simulink model "solics_inverter_model_updated"  (R2024a)
settings: Solver=VariableStepAuto  StartTime=0.0  StopTime=1  RelTol=1e-3
libraries: spsSeriesRLCBranchLib x7, spsIGBTLib x5, spsVoltageMeasurementLib x4, spsCurrentMeasurementLib x3, spsGroundLib x2, spsDiodeLib x1, spsPVArrayLib x1, spsPWMGeneratorDCDCLib x1, spsTriangleGeneratorLib x1, spspowerguiLib x1
settings Model: Creator=dogba  LastModifiedBy=dogba

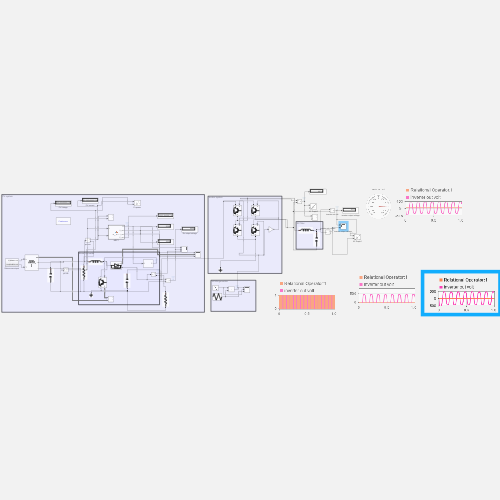
[thumbnail: Simulink's stored preview of the top-level diagram]
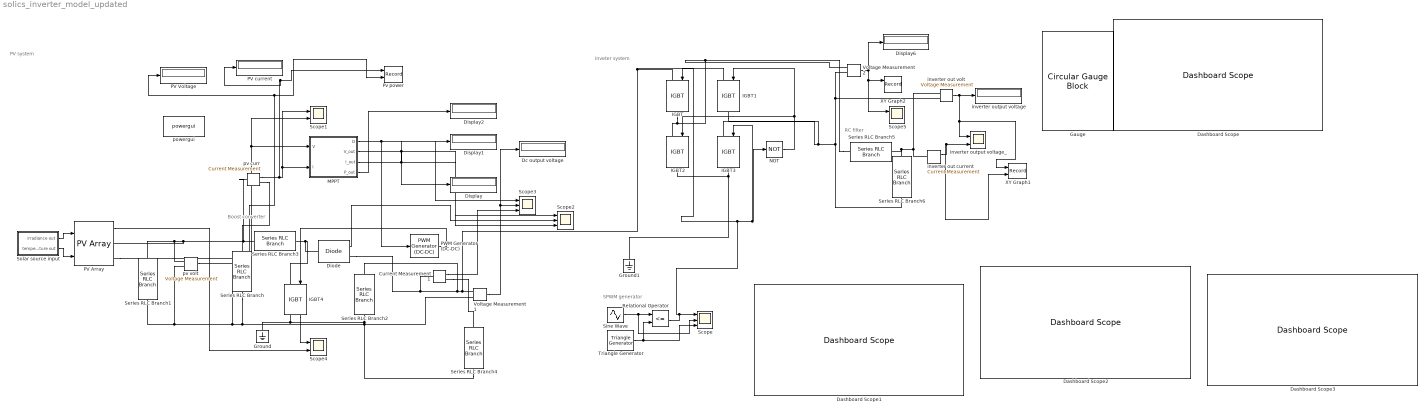
== system solics_inverter_model_updated ==
  note: inveter system
  note: RC filter
  note: Boost converter
  note: SPWM generator
  note: PV system
  Current Measurement1 : spsCurrentMeasurementLib/Current Measurement  PhasorSimulation=off  OutputType=Complex  PSBequivalent=0
  Dashboard Scope{,1..3} (4 alike) : DashboardScope  Ymin=-500  Ymax=500
  Dc output voltage : Display
  Diode : spsDiodeLib/Diode  Ron=0.001  Lon=0  Vf=0.8  IC=0  UseSnubber=0  Rs=500  Cs=250e-9  Measurements=on
  Display{,1..2,6} (4 alike) : Display
      Display2 settings: Format=decimal (Stored Integer)  Decimation=4
  Gauge : CircularGaugeBlock  ScaleMin=-500  ScaleMax=500
  Ground : spsGroundLib/Ground  LConnTagsString=a
  Ground1 : spsGroundLib/Ground  LConnTagsString=a
  IGBT{,1..3} (4 alike) : spsIGBTLib/IGBT  Ron=0.001  Lon=0  Vf=1  Tf=1e-6  Tt=2e-6  IC=0  Rs=1e5  Cs=inf  Measurements=off
  IGBT4 : spsIGBTLib/IGBT  Ron=0.001  Lon=0  Vf=1  Tf=1e-6  Tt=2e-6  IC=0  Rs=1e5  Cs=inf  Measurements=on
  MPPT : MATLAB Function  TreatAsAtomicUnit=on  SystemSampleTime=1e-4
  NOT : Logic  Operator=NOT  IconShape=distinctive  AllPortsSameDT=off  OutDataTypeStr=boolean
  PV Array : spsPVArrayLib/PV Array  Npar=40  Nser=10  PlotType=array @ 1000 W/m2 & specified temperatures  S_vec="[ 1000  500  100 ]"  Temp_C_vec="[ 45 25  ]"  ModuleName=User-defined  PlotWhenSelected=off  Pm=213.15  Ncell=60  Voc=36.3  Isc=7.84  Vm=29  Im=7.35  beta_Voc_pc=-0.36099  alpha_Isc_pc=0.102  beta_Voc=-0.13104  alpha_Isc=0.0079968  IL=7.8654  I0=2.9273e-10  nI=0.98119  Rsh=313.0553  Rs=0.39381  RobustModel=off  RobustCellTemperature=313.3991  BAL=on  Tc=1e-6  Tfilter=5e-5
  PV Voltage : Display
      settings: Format=decimal (Stored Integer)  Decimation=4
  PV current : Display
      settings: Format=decimal (Stored Integer)  Decimation=4
  PWM Generator (DC-DC) : spsPWMGeneratorDCDCLib/PWM Generator (DC-DC)  Fsw=20e3  Ts=1e-5
  Pv power : Record  FileSettingsInternal="{\"entries\":[{\"content\":{\"excelSettings\":{\"content\":{},\"type\":\"Streamout.ExcelSettings\"}},\"type\":\"Streamout.FileSettingStorage\",\"uuid\":\"\"}],\"packageUris\":[\"http:\\/\\/schema.mathworks.com\\/mf0\\/streamout_blocks\\/R2020a\"],\"version\":\"1.0\"}"  Layout=[1 1]  SignalsInternal="{\"entries\":[{\"content\":{\"signals\":[{\"content\":{\"blockPath\":[],\"dimensions\":[1],\"domain\":\"\",\"lineColor\":\"#a2142f\",\"plots\":[ 1 ],\"port\":1,\"sid\":[\"\"],\"signalID\":1,\"signalName\":\"pv curr\"},\"type\":\"RecordBlkView.Signal\",\"uuid\":\"\"},{\"content\":{\"blockPath\":[],\"dimensions\":[1],\"domain\":\"\",\"lineColor\":\"#139fff\",\"plots\":[ 1 ],\"port\":2,\"sid\":[\"\"],\"signalID\":2,\"signalName\":\"pv volt\"},\"type\":\"RecordBlkView.Signal\",\"uuid\":\"\"}]},\"type\":\"RecordBlkView.InputSignals\",\"uuid\":\"\"}],\"packageUris\":[\"http:\\/\\/schema.mathworks.com\\/mf0\\/streamout_blocks\\/R2020a\"],\"version\":\"1.0\"}"  VisualizationBindings="{\"xyplotplugin\":{\"info\":[{\"series\":[{\"bindingParametersList\":[{\"parameter\":\"X-Axis\",\"signalID\":1,\"signalName\":\"pv curr\"},{\"parameter\":\"Y-Axis\",\"signalID\":2,\"signalName\":\"pv volt\"},{\"parameter\":\"X-Axis\",\"signalID\":1,\"signalName\":\"pv curr\"},{\"parameter\":\"Y-Axis\",\"signalID\":2,\"signalName\":\"pv volt\"}],\"seriesID\":0}],\"subplotID\":1}]}}"  CompatibilityTag=XY
  Relational Operator : RelationalOperator  Operator=<=  OutDataTypeStr=boolean  RndMeth=Simplest  InputSameDT=off
  Scope : Scope  NumInputPorts=3
  Scope1 : Scope  NumInputPorts=2
  Scope2 : Scope  NumInputPorts=3
  Scope3 : Scope  NumInputPorts=3
  Scope4 : Scope  NumInputPorts=2
  Scope5 : Scope  NumInputPorts=2
  Series RLC Branch : spsSeriesRLCBranchLib/Series RLC Branch  LConnTagsString=__new0  RConnTagsString=__new0  BranchType=R  Resistance=10  Inductance=1e-3  SetiL0=off  InitialCurrent=0  Capacitance=1e-6  Setx0=off  InitialVoltage=0  Measurements=None
  Series RLC Branch1 : spsSeriesRLCBranchLib/Series RLC Branch  LConnTagsString=__new0  RConnTagsString=__new0  BranchType=C  Resistance=10  Inductance=1e-3  SetiL0=off  InitialCurrent=0  Capacitance=1e-6  Setx0=off  InitialVoltage=0  Measurements=None
  Series RLC Branch2 : spsSeriesRLCBranchLib/Series RLC Branch  LConnTagsString=__new0  RConnTagsString=__new0  BranchType=C  Resistance=10  Inductance=1e-3  SetiL0=off  InitialCurrent=0  Capacitance=1000e-6  Setx0=off  InitialVoltage=0  Measurements=None
  Series RLC Branch3 : spsSeriesRLCBranchLib/Series RLC Branch  LConnTagsString=__new0  RConnTagsString=__new0  BranchType=L  Resistance=10  Inductance=2e-3  SetiL0=off  InitialCurrent=0  Capacitance=1e-6  Setx0=off  InitialVoltage=0  Measurements=None
  Series RLC Branch4 : spsSeriesRLCBranchLib/Series RLC Branch  LConnTagsString=__new0  RConnTagsString=__new0  BranchType=R  Resistance=50  Inductance=1e-3  SetiL0=off  InitialCurrent=0  Capacitance=1e-6  Setx0=off  InitialVoltage=0  Measurements=None
  Series RLC Branch5 : spsSeriesRLCBranchLib/Series RLC Branch  LConnTagsString=__new0  RConnTagsString=__new0  BranchType=L  Resistance=50  Inductance=10e-3  SetiL0=off  InitialCurrent=0  Capacitance=1e-6  Setx0=off  InitialVoltage=0  Measurements=None
  Series RLC Branch6 : spsSeriesRLCBranchLib/Series RLC Branch  LConnTagsString=__new0  RConnTagsString=__new0  BranchType=C  Resistance=50  Inductance=5e-3  SetiL0=off  InitialCurrent=0  Capacitance=10e-6  Setx0=off  InitialVoltage=0  Measurements=None
  Sine Wave : Sin  Frequency=50  SampleTime=0
  Solar source input : Subsystem
  Triangle Generator : spsTriangleGeneratorLib/Triangle Generator  Freq=10e3  Phase=90  Ts=0
  Voltage Measurement1 : spsVoltageMeasurementLib/Voltage Measurement  PhasorSimulation=off  OutputType=Complex  PSBequivalent=0
  Voltage Measurement2 : spsVoltageMeasurementLib/Voltage Measurement  PhasorSimulation=off  OutputType=Complex  PSBequivalent=0
  XY Graph1 : Record  FileSettingsInternal="{\"entries\":[{\"content\":{\"excelSettings\":{\"content\":{},\"type\":\"Streamout.ExcelSettings\"}},\"type\":\"Streamout.FileSettingStorage\",\"uuid\":\"\"}],\"packageUris\":[\"http:\\/\\/schema.mathworks.com\\/mf0\\/streamout_blocks\\/R2020a\"],\"version\":\"1.0\"}"  Layout=[1 1]  SignalsInternal="{\"entries\":[{\"content\":{\"signals\":[{\"content\":{\"blockPath\":[],\"dimensions\":[1],\"domain\":\"\",\"lineColor\":\"#ff13a6\",\"lineWidth\":2,\"port\":1,\"sid\":[\"\"],\"signalID\":1,\"signalName\":\"inverter out volt\"},\"type\":\"RecordBlkView.Signal\",\"uuid\":\"\"},{\"content\":{\"blockPath\":[],\"dimensions\":[1],\"domain\":\"\",\"lineColor\":\"#fe330a\",\"lineWidth\":2,\"port\":2,\"sid\":[\"\"],\"signalID\":2,\"signalName\":\"inverter out current\"},\"type\":\"RecordBlkView.Signal\",\"uuid\":\"\"}]},\"type\":\"RecordBlkView.InputSignals\",\"uuid\":\"\"}],\"packageUris\":[\"http:\\/\\/schema.mathworks.com\\/mf0\\/streamout_blocks\\/R2020a\"],\"version\":\"1.0\"}"  VisualizationBindings="{\"xyplotplugin\":{\"info\":[{\"series\":[],\"subplotID\":1}]}}"  CompatibilityTag=XY
  XY Graph2 : Record  FileSettingsInternal="{\"entries\":[{\"content\":{\"excelSettings\":{\"content\":{},\"type\":\"Streamout.ExcelSettings\"}},\"type\":\"Streamout.FileSettingStorage\",\"uuid\":\"\"}],\"packageUris\":[\"http:\\/\\/schema.mathworks.com\\/mf0\\/streamout_blocks\\/R2020a\"],\"version\":\"1.0\"}"  Layout=[1 1]  SignalsInternal="{\"entries\":[{\"content\":{\"signals\":[{\"content\":{\"blockPath\":[],\"dimensions\":[1],\"domain\":\"\",\"lineColor\":\"#139fff\",\"lineWidth\":2,\"port\":1,\"sid\":[\"\"],\"signalID\":1,\"signalName\":\"Voltage Measurement2\"},\"type\":\"RecordBlkView.Signal\",\"uuid\":\"\"},{\"content\":{\"blockPath\":[],\"dimensions\":[1],\"domain\":\"\",\"lineColor\":\"#22b573\",\"lineWidth\":2,\"port\":2,\"sid\":[\"\"],\"signalID\":2},\"type\":\"RecordBlkView.Signal\",\"uuid\":\"\"}]},\"type\":\"RecordBlkView.InputSignals\",\"uuid\":\"\"}],\"packageUris\":[\"http:\\/\\/schema.mathworks.com\\/mf0\\/streamout_blocks\\/R2020a\"],\"version\":\"1.0\"}"  VisualizationBindings="{\"xyplotplugin\":{\"info\":[{\"series\":[],\"subplotID\":1}]}}"  CompatibilityTag=XY
  inverter out current : spsCurrentMeasurementLib/Current Measurement  PhasorSimulation=off  OutputType=Complex  PSBequivalent=0
  inverter out volt : spsVoltageMeasurementLib/Voltage Measurement  PhasorSimulation=off  OutputType=Complex  PSBequivalent=0
  inverter output voltage : Display
  inverter output voltage_ : Scope  NumInputPorts=2
  powergui : spspowerguiLib/powergui  Priority=1  SimulationMode=Continuous  SampleTime=50e-6  frequency=60  Iterations=50  frequencyindice=0  Pbase=100e6  ErrMax=1e-4  UnitsV=kV  UnitsW=MW  buscounter=0  FunctionMessages=off  echomessages=off  EnableUseOfTLC=off  CurrentSourceSwitches=off  DisableSnubberDevices=off  DisableRonSwitches=off  DisableVfSwitches=off  DisplayEquations=off  AutomaticDiscreteSolvers=off  SolverType=Tustin/Backward Euler (TBE)  Interpol=off  ExternalGateDelay=off  methode=off  Ts=100  x0status=blocks  SPID=on  SwTol=0  HookPort=off  NonlinearTolerance=1e-4  nMaxIteration=100  ContinueOnMaxIteration=off  RestoreLinks=warning  ResistiveCurrentMeasurement=off  Frange=[0:2:500]  Ylog=off  Xlog=on  ShowGrid=off  save=off  variable=ZData  structure=0  ZoomFFT=off  StartTime=0.0  cycles=1  DisplayStyle=1  fundamental=60  FreqAxis=off  MaxFrequency=1000  frequencyindicesteady=1  RmsSteady=1  display=off
  pv curr : spsCurrentMeasurementLib/Current Measurement  PhasorSimulation=off  OutputType=Complex  PSBequivalent=0
  pv volt : spsVoltageMeasurementLib/Voltage Measurement  PhasorSimulation=off  OutputType=Complex  PSBequivalent=0
  wires:
  Voltage Measurement1/1 -> Dc output voltage/1, Scope3/2
  pv volt/1 -> Scope1/2, MPPT/1(V), Pv power/2, PV Voltage/1
  MPPT/3(I_out) -> Display1/1, Scope2/1
  Solar source input/2(temperature out) -> PV Array/2
  pv curr/1 -> Scope1/1, MPPT/2(I), Pv power/1, PV current/1
  Solar source input/1(irradiance out) -> PV Array/1
  MPPT/4(P_out) -> Display2/1
  MPPT/2(V_out) -> Display/1, Scope2/3
  Sine Wave/1 -> Scope/2, Relational Operator/1
  Triangle Generator/1 -> Scope/3, Relational Operator/2
  Current Measurement1/1 -> Scope3/3
  Diode/1 -> Scope2/2
  MPPT/1(D) -> PWM Generator (DC-DC)/1, Scope3/1
  PV Array/1 -> Scope4/2
  IGBT4/1 -> Scope4/1
  PWM Generator (DC-DC)/1 -> IGBT4/1
  Voltage Measurement2/1 -> XY Graph2/1, Scope5/1, Display6/1
  inverter out volt/1 -> inverter output voltage/1, inverter output voltage_/1, XY Graph1/1
  NOT/1 -> IGBT1/1, IGBT2/1
  Relational Operator/1 -> IGBT/1, IGBT3/1, NOT/1, Scope/1
  inverter out current/1 -> inverter output voltage_/2, XY Graph1/2
  connections:
  IGBT/LConn1 -- Voltage Measurement1/LConn1 -- Diode/RConn1 -- Current Measurement1/LConn1 -- Series RLC Branch2/LConn1 -- IGBT1/LConn1
  Series RLC Branch1/LConn1 -- pv volt/LConn1 -- Series RLC Branch3/LConn1 -- pv curr/LConn1 -- PV Array/RConn1
  pv volt/LConn2 -- PV Array/RConn2 -- Series RLC Branch/RConn1 -- Series RLC Branch4/RConn1 -- Voltage Measurement1/LConn2 -- Ground/LConn1 -- IGBT4/RConn1 -- Series RLC Branch2/RConn1 -- Series RLC Branch1/RConn1
  Current Measurement1/RConn1 -- Series RLC Branch4/LConn1
  pv curr/RConn1 -- Series RLC Branch/LConn1
  IGBT4/LConn1 -- Diode/LConn1 -- Series RLC Branch3/RConn1
  Series RLC Branch6/LConn1 -- inverter out volt/LConn1 -- inverter out current/LConn1 -- Series RLC Branch5/RConn1
  inverter out volt/LConn2 -- Voltage Measurement2/LConn2 -- IGBT1/RConn1 -- IGBT3/LConn1 -- Series RLC Branch6/RConn1
  Series RLC Branch5/LConn1 -- Voltage Measurement2/LConn1 -- IGBT/RConn1 -- IGBT2/LConn1
  IGBT2/RConn1 -- IGBT3/RConn1 -- Ground1/LConn1

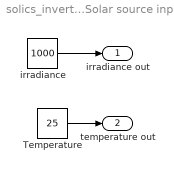
== system solics_inverter_model_updated/Solar source input ==
  Temperature : Constant  Value=25
  irradiance : Constant  Value=1000
  irradiance out : Outport
  temperature out : Outport  Port=2
  wires:
  irradiance/1 -> irradiance out/1
  Temperature/1 -> temperature out/1

== matlab function solics_inverter_model_updated/MPPT ==
  data: V input; D output; I input; V_out output; I_out output; P_out output
function [D, V_out, I_out, P_out] = PO_MPPT(V, I)

% Persistent variables to store previous values
persistent V_prev I_prev P_prev D_prev

if isempty(V_prev)
    V_prev = 0;
    I_prev = 0;
    P_prev = 0;
    D_prev = 0.5; % Start at middle
end

% Compute power
P = V * I;
dP = P - P_prev;
dV = V - V_prev;

% Perturb and Observe Logic
if dP ~= 0
    if dP > 0
        if dV > 0
            D_prev = D_prev - 0.01;
        else
            D_prev = D_prev + 0.01;
        end
    else
        if dV > 0
            D_prev = D_prev + 0.01;
        else
            D_prev = D_prev - 0.01;
        end
    end
end

% Clamp duty cycle between 0.1 and 0.9
D = max(0.1, min(0.9, D_prev));

% Update past values
V_prev = V;
I_prev = I;
P_prev = P;

% For debugging
V_out = V;
I_out = I;
P_out = P;
